simulink model "bscfsm"  (R2016a)
settings: Solver=FixedStepAuto  StartTime=0.0  StopTime=10  RelTol=1e-3
model workspace (MAT data in the model file):
  F = [0; 0; 0; 0; 0; 0; 0; 0; 0; 0; 0; 0; 0; 0; 0; 0; 0; 0; 0; 0; 0; 0; 0; 0; 0; 0; 0; 0; 0; 0; 0; 0; 0; 0; 0; 0; 0; 0; 0; 0; 0; 0; 0; 0; 0; 0; 0; 0; 0; 0; 0]
  FR = [0; 0; 0; 0; 0; 0]
  Ft = 0
  InputSize = 6
  M = [0 0 0 1 1 0 3 5.8]
  N = 32
  T = table
  T.nrows = 1
  T.nvars = 8
  T.varnames = {'Var1', 'Var2', 'Var3', 'Var4', 'Var5', 'Var6', 'Var7', 'Var8'}
  T.data = {0, 0, 0, 1, 1, 0, 3, 5.8}
  TimeSteps = 51
  X = [0 1 0 1 1 0 1 0 0.988521387031 1 1 0.0114786129688 ... (1224 elements, 6x204)]
  apfail = [0; 1; 0; 0.995818544823; 0; 0; 1; 0.00917624141749; 0.992109239838; 0; 0; 0.0226449188505; 0; 1; 1; 0; 0; 0.969073769871; 0; 0; 1; 0; 1; 1; 0.964844416339; 0; 1; 0; 0; 0; 1; 0; 0.982847610626; 1; 1; 1; 1; 1; 0; 1; 0; 1; 1; 0; 0.958770144702; 1; 1; 0; 1; 1; 0]
  cs : Simulink.ConfigSet (value not decoded)
  curPath = ''
  d = 52
  good = [0; 1; 1; 1; 1; 1; 1; 1; 1; 1; 1; 1; 1; 1; 1; 1; 1; 1; 1; 1; 1; 1; 1; 1; 1; 1; 1; 1; 1; 1; 1; 1; 1; 1; 1; 1; 1; 1; 1; 1; 1; 1; 1; 1; 1; 1; 1; 1; 1; 1; 1]
  hws : Simulink.ModelWorkspace (value not decoded)
  i = 14
  j = 51
  limits = [1; 0; 0; 0; 0; 0; 0; 1; 0; 1; 0.00163106788269; 1; 1; 1; 1; 0; 1; 0; 0; 1; 1; 0.0696477276458; 1; 1; 1; 0; 1; 0; 1; 1; 1; 0; 0.98345473187; 1; 0; 1; 1; 0.00166422824427; 0; 0; 1; 1; 0; 1; 0; 0; 0; 1; 0; 1; 1]
  list(1).name = 'F'
  list(1).size = [51 1]
  list(1).bytes = 408
  list(1).class = 'double'
  list(1).global = 0
  list(1).sparse = 0
  list(1).complex = 0
  list(1).nesting.function = 'simfsm'
  list(1).nesting.level = 1
  list(1).persistent = 0
  list(2).name = 'FR'
  list(2).size = [6 1]
  list(2).bytes = 48
  list(2).class = 'double'
  list(2).global = 0
  list(2).sparse = 0
  list(2).complex = 0
  list(2).nesting.function = 'simfsm'
  list(2).nesting.level = 1
  list(2).persistent = 0
  list(3).name = 'Ft'
  list(3).size = [1 1]
  list(3).bytes = 8
  list(3).class = 'double'
  list(3).global = 0
  list(3).sparse = 0
  list(3).complex = 0
  list(3).nesting.function = 'simfsm'
  list(3).nesting.level = 1
  list(3).persistent = 0
  list(4).name = 'InputSize'
  list(4).size = [1 1]
  list(4).bytes = 8
  list(4).class = 'double'
  list(4).global = 0
  list(4).sparse = 0
  list(4).complex = 0
  list(4).nesting.function = 'simfsm'
  list(4).nesting.level = 1
  list(4).persistent = 0
  list(5).name = 'N'
  list(5).size = [1 1]
  list(5).bytes = 8
  list(5).class = 'double'
  list(5).global = 0
  list(5).sparse = 0
  list(5).complex = 0
  list(5).nesting.function = 'simfsm'
  list(5).nesting.level = 1
  list(5).persistent = 0
  list(6).name = 'TimeSteps'
  list(6).size = [1 1]
  list(6).bytes = 8
  list(6).class = 'double'
  list(6).global = 0
  list(6).sparse = 0
  list(6).complex = 0
  list(6).nesting.function = 'simfsm'
  list(6).nesting.level = 1
  list(6).persistent = 0
  list(7).name = 'X'
  list(7).size = [6 204]
  list(7).bytes = 9792
  list(7).class = 'double'
  list(7).global = 0
  list(7).sparse = 0
  list(7).complex = 0
  list(7).nesting.function = 'simfsm'
  list(7).nesting.level = 1
  list(7).persistent = 0
  list(8).name = 'apfail'
  list(8).size = [51 1]
  list(8).bytes = 408
  list(8).class = 'double'
  list(8).global = 0
  list(8).sparse = 0
  list(8).complex = 0
  list(8).nesting.function = 'simfsm'
  list(8).nesting.level = 1
  list(8).persistent = 0
  list(9).name = 'cs'
  list(9).size = [1 1]
  list(9).bytes = 0
  list(9).class = 'Simulink.ConfigSet'
  list(9).global = 0
  list(9).sparse = 0
  list(9).complex = 0
  list(9).nesting.function = 'simfsm'
  list(9).nesting.level = 1
  list(9).persistent = 0
  list(10).name = 'curPath'
  list(10).size = [0 0]
  list(10).bytes = 0
  list(10).class = 'char'
  list(10).global = 0
  list(10).sparse = 0
  list(10).complex = 0
  list(10).nesting.function = 'simfsm'
  list(10).nesting.level = 1
  list(10).persistent = 0
  list(11).name = 'd'
  list(11).size = [1 1]
  list(11).bytes = 8
  list(11).class = 'double'
  list(11).global = 0
  list(11).sparse = 0
  list(11).complex = 0
  list(11).nesting.function = 'simfsm'
  list(11).nesting.level = 1
  list(11).persistent = 0
  list(12).name = 'good'
  list(12).size = [51 1]
  list(12).bytes = 51
  list(12).class = 'logical'
  list(12).global = 0
  list(12).sparse = 0
  list(12).complex = 0
  list(12).nesting.function = 'simfsm'
  list(12).nesting.level = 1
  list(12).persistent = 0
  list(13).name = 'hws'
  list(13).size = [1 1]
  list(13).bytes = 0
  list(13).class = 'Simulink.ModelWorkspace'
  list(13).global = 0
  list(13).sparse = 0
  list(13).complex = 0
  list(13).nesting.function = 'simfsm'
  list(13).nesting.level = 1
  list(13).persistent = 0
  list(14).name = 'i'
  list(14).size = [1 1]
  list(14).bytes = 8
  list(14).class = 'double'
  list(14).global = 0
  list(14).sparse = 0
  list(14).complex = 0
  list(14).nesting.function = 'simfsm'
  list(14).nesting.level = 1
  list(14).persistent = 0
  list(15).name = 'j'
  list(15).size = [1 1]
  list(15).bytes = 8
  list(15).class = 'double'
  list(15).global = 0
  list(15).sparse = 0
  list(15).complex = 0
  list(15).nesting.function = 'simfsm'
  list(15).nesting.level = 1
  list(15).persistent = 0
  list(16).name = 'limits'
  list(16).size = [51 1]
  list(16).bytes = 408
  list(16).class = 'double'
  list(16).global = 0
  list(16).sparse = 0
  list(16).complex = 0
  list(16).nesting.function = 'simfsm'
  list(16).nesting.level = 1
  list(16).persistent = 0
  list(17).name = 'list'
  list(17).size = [32 1]
  list(17).bytes = 46434
  list(17).class = 'struct'
  list(17).global = 0
  list(17).sparse = 0
  list(17).complex = 0
  list(17).nesting.function = 'simfsm'
  list(17).nesting.level = 1
  list(17).persistent = 0
  list(18).name = 'mode'
  list(18).size = [51 1]
  list(18).bytes = 51
  list(18).class = 'logical'
  list(18).global = 0
  list(18).sparse = 0
  list(18).complex = 0
  list(18).nesting.function = 'simfsm'
  list(18).nesting.level = 1
  list(18).persistent = 0
  list(19).name = 'model_cs'
  list(19).size = [1 1]
  list(19).bytes = 0
  list(19).class = 'Simulink.ConfigSet'
  list(19).global = 0
  list(19).sparse = 0
  list(19).complex = 0
  list(19).nesting.function = 'simfsm'
  list(19).nesting.level = 1
  list(19).persistent = 0
  list(20).name = 'modelpath'
  list(20).size = [0 0]
  list(20).bytes = 0
  list(20).class = 'char'
  list(20).global = 0
  list(20).sparse = 0
  list(20).complex = 0
  list(20).nesting.function = 'simfsm'
  list(20).nesting.level = 1
  list(20).persistent = 0
  list(21).name = 'n'
  list(21).size = [1 1]
  list(21).bytes = 8
  list(21).class = 'double'
  list(21).global = 0
  list(21).sparse = 0
  list(21).complex = 0
  list(21).nesting.function = 'simfsm'
  list(21).nesting.level = 1
  list(21).persistent = 0
  list(22).name = 'nbrInputs'
  list(22).size = [1 1]
  list(22).bytes = 8
  list(22).class = 'double'
  list(22).global = 0
  list(22).sparse = 0
  list(22).complex = 0
  list(22).nesting.function = 'simfsm'
  list(22).nesting.level = 1
  list(22).persistent = 0
  list(23).name = 'pullup'
  list(23).size = [51 1]
  list(23).bytes = 51
  list(23).class = 'logical'
  list(23).global = 0
  list(23).sparse = 0
  list(23).complex = 0
  list(23).nesting.function = 'simfsm'
  list(23).nesting.level = 1
  list(23).persistent = 0
  list(24).name = 'request'
  list(24).size = [51 1]
  list(24).bytes = 51
  list(24).class = 'logical'
  list(24).global = 0
  list(24).sparse = 0
  list(24).complex = 0
  list(24).nesting.function = 'simfsm'
  list(24).nesting.level = 1
  list(24).persistent = 0
  list(25).name = 'senstate'
  list(25).size = [51 1]
  list(25).bytes = 408
  list(25).class = 'double'
  list(25).global = 0
  list(25).sparse = 0
  list(25).complex = 0
  list(25).nesting.function = 'simfsm'
  list(25).nesting.level = 1
  list(25).persistent = 0
  list(26).name = 'simOut'
  list(26).size = [1 1]
  list(26).bytes = 34272
  list(26).class = 'Simulink.SimulationOutput'
  list(26).global = 0
  list(26).sparse = 0
  list(26).complex = 0
  list(26).nesting.function = 'simfsm'
  list(26).nesting.level = 1
  list(26).persistent = 0
  list(27).name = 'standby'
  list(27).size = [51 1]
  list(27).bytes = 408
  list(27).class = 'double'
  list(27).global = 0
  list(27).sparse = 0
  list(27).complex = 0
  list(27).nesting.function = 'simfsm'
  list(27).nesting.level = 1
  list(27).persistent = 0
  list(28).name = 'state'
  list(28).size = [51 1]
  list(28).bytes = 408
  list(28).class = 'double'
  list(28).global = 0
  list(28).sparse = 0
  list(28).complex = 0
  list(28).nesting.function = 'simfsm'
  list(28).nesting.level = 1
  list(28).persistent = 0
  list(29).name = 'supported'
  list(29).size = [51 1]
  list(29).bytes = 408
  list(29).class = 'double'
  list(29).global = 0
  list(29).sparse = 0
  list(29).complex = 0
  list(29).nesting.function = 'simfsm'
  list(29).nesting.level = 1
  list(29).persistent = 0
  list(30).name = 't'
  list(30).size = [51 1]
  list(30).bytes = 408
  list(30).class = 'double'
  list(30).global = 0
  list(30).sparse = 0
  list(30).complex = 0
  list(30).nesting.function = 'simfsm'
  list(30).nesting.level = 1
  list(30).persistent = 0
  list(31).name = 'var'
  list(31).size = [1 1]
  list(31).bytes = 3448
  list(31).class = 'struct'
  list(31).global = 0
  list(31).sparse = 0
  list(31).complex = 0
  list(31).nesting.function = 'simfsm'
  list(31).nesting.level = 1
  list(31).persistent = 0
  list(32).name = 'varout'
  list(32).size = [1 1]
  list(32).bytes = 4924
  list(32).class = 'struct'
  list(32).global = 0
  list(32).sparse = 0
  list(32).complex = 0
  list(32).nesting.function = 'simfsm'
  list(32).nesting.level = 1
  list(32).persistent = 0
  mode = [1; 1; 0; 1; 0; 1; 1; 0; 0; 1; 1; 1; 1; 1; 1; 1; 1; 1; 1; 0; 1; 1; 1; 1; 1; 1; 1; 1; 1; 1; 1; 1; 1; 1; 1; 1; 1; 1; 1; 1; 1; 1; 1; 0; 1; 1; 1; 1; 1; 1; 1]
  model_cs : Simulink.ConfigSet (value not decoded)
  modelpath = ''
  n = 6
  nbrInputs = 4
  nbrelements = 204
  pullup = [0; 1; 0; 0; 0; 0; 1; 0; 0; 0; 0; 1; 0; 1; 0; 0; 0; 1; 0; 0; 0; 0; 1; 0; 1; 1; 0; 0; 0; 1; 0; 1; 0; 1; 0; 1; 0; 1; 0; 1; 1; 0; 1; 0; 0; 1; 1; 1; 0; 1; 0]
  request = [0; 0; 1; 0; 1; 0; 0; 1; 1; 0; 0; 0; 0; 0; 0; 0; 0; 0; 0; 1; 0; 0; 0; 0; 0; 0; 0; 0; 0; 0; 0; 0; 0; 0; 0; 0; 0; 0; 0; 0; 0; 0; 0; 1; 0; 0; 0; 0; 0; 0; 0]
  senstate = [2; 1; 1; 1; 1; 1; 1; 1; 1; 1; 1; 1; 1; 1; 1; 1; 1; 1; 1; 1; 1; 1; 1; 1; 1; 1; 1; 1; 1; 1; 1; 1; 1; 1; 1; 1; 1; 1; 1; 1; 1; 1; 1; 1; 1; 1; 1; 1; 1; 1; 1]
  simOut = Simulink.SimulationOutput
  simOut.Data.tout = [0; 0.2; 0.4; 0.6; 0.8; 1; 1.2; 1.4; 1.6; 1.8; 2; 2.2; 2.4; 2.6; 2.8; 3; 3.2; 3.4; 3.6; 3.8; 4; 4.2; 4.4; 4.6; 4.8; 5; 5.2; 5.4; 5.6; 5.8; 6; 6.2; 6.4; 6.6; 6.8; 7; 7.2; 7.4; 7.6; 7.8; 8; 8.2; 8.4; 8.6; 8.8; 9; 9.2; 9.4; 9.6; 9.8; 10]
  simOut.Data.varout.time = [0; 0.2; 0.4; 0.6; 0.8; 1; 1.2; 1.4; 1.6; 1.8; 2; 2.2; 2.4; 2.6; 2.8; 3; 3.2; 3.4; 3.6; 3.8; 4; 4.2; 4.4; 4.6; 4.8; 5; 5.2; 5.4; 5.6; 5.8; 6; 6.2; 6.4; 6.6; 6.8; 7; 7.2; 7.4; 7.6; 7.8; 8; 8.2; 8.4; 8.6; 8.8; 9; 9.2; 9.4; 9.6; 9.8; 10]
  simOut.Data.varout.signals(1).values = [0; 1; 0; 0; 0; 0; 1; 0; 0; 0; 0; 1; 0; 1; 0; 0; 0; 1; 0; 0; 0; 0; 1; 0; 1; 1; 0; 0; 0; 1; 0; 1; 0; 1; 0; 1; 0; 1; 0; 1; 1; 0; 1; 0; 0; 1; 1; 1; 0; 1; 0]
  simOut.Data.varout.signals(1).dimensions = 1
  simOut.Data.varout.signals(1).label = ''
  simOut.Data.varout.signals(1).blockName = 'bscfsm/pullup'
  simOut.Data.varout.signals(2).values = [3; 2; 0; 3; 0; 3; 2; 0; 0; 3; 3; 2; 3; 2; 3; 3; 3; 2; 3; 0; 3; 3; 2; 3; 2; 2; 3; 3; 3; 2; 3; 2; 3; 2; 3; 2; 3; 2; 3; 2; 2; 3; 2; 0; 3; 2; 2; 2; 3; 2; 3]
  simOut.Data.varout.signals(2).dimensions = 1
  simOut.Data.varout.signals(2).label = ''
  simOut.Data.varout.signals(2).blockName = 'bscfsm/state'
  simOut.Data.varout.signals(3).values = [0; 1; 1; 1; 1; 1; 1; 1; 1; 1; 1; 1; 1; 1; 1; 1; 1; 1; 1; 1; 1; 1; 1; 1; 1; 1; 1; 1; 1; 1; 1; 1; 1; 1; 1; 1; 1; 1; 1; 1; 1; 1; 1; 1; 1; 1; 1; 1; 1; 1; 1]
  simOut.Data.varout.signals(3).dimensions = 1
  simOut.Data.varout.signals(3).label = ''
  simOut.Data.varout.signals(3).blockName = 'bscfsm/good'
  simOut.Data.varout.signals(4).values = [2; 1; 1; 1; 1; 1; 1; 1; 1; 1; 1; 1; 1; 1; 1; 1; 1; 1; 1; 1; 1; 1; 1; 1; 1; 1; 1; 1; 1; 1; 1; 1; 1; 1; 1; 1; 1; 1; 1; 1; 1; 1; 1; 1; 1; 1; 1; 1; 1; 1; 1]
  simOut.Data.varout.signals(4).dimensions = 1
  simOut.Data.varout.signals(4).label = ''
  simOut.Data.varout.signals(4).blockName = 'bscfsm/SENSTATE'
  simOut.Data.varout.signals(5).values = [1; 1; 0; 1; 0; 1; 1; 0; 0; 1; 1; 1; 1; 1; 1; 1; 1; 1; 1; 0; 1; 1; 1; 1; 1; 1; 1; 1; 1; 1; 1; 1; 1; 1; 1; 1; 1; 1; 1; 1; 1; 1; 1; 0; 1; 1; 1; 1; 1; 1; 1]
  simOut.Data.varout.signals(5).dimensions = 1
  simOut.Data.varout.signals(5).label = ''
  simOut.Data.varout.signals(5).blockName = 'bscfsm/MODE'
  simOut.Data.varout.signals(6).values = [0; 0; 1; 0; 1; 0; 0; 1; 1; 0; 0; 0; 0; 0; 0; 0; 0; 0; 0; 1; 0; 0; 0; 0; 0; 0; 0; 0; 0; 0; 0; 0; 0; 0; 0; 0; 0; 0; 0; 0; 0; 0; 0; 1; 0; 0; 0; 0; 0; 0; 0]
  simOut.Data.varout.signals(6).dimensions = 1
  simOut.Data.varout.signals(6).label = ''
  simOut.Data.varout.signals(6).blockName = 'bscfsm/REQUEST'
  simOut.Metadata = Simulink.SimulationMetadata
  simOut.Metadata.ModelInfo.ModelName = 'bscfsm'
  simOut.Metadata.ModelInfo.ModelVersion = '1.101'
  simOut.Metadata.ModelInfo.ModelFilePath = '/Users/ceren.gebizli/Desktop/Shiva/QRA-Search/QRA-Search/SimulinkModels/1_fsm/bscfsm.slx'
  simOut.Metadata.ModelInfo.UserID = 'ceren.gebizli'
  simOut.Metadata.ModelInfo.MachineName = ''
  simOut.Metadata.ModelInfo.Platform = 'MACI64'
  simOut.Metadata.ModelInfo.ModelStructuralChecksum = [2182324134; 966261521; 1592501320; 2819510478]
  simOut.Metadata.ModelInfo.SimulationMode = 'normal'
  simOut.Metadata.ModelInfo.StartTime = 0
  simOut.Metadata.ModelInfo.StopTime = 10
  simOut.Metadata.ModelInfo.SolverInfo.Type = 'Fixed-Step'
  simOut.Metadata.ModelInfo.SolverInfo.Solver = 'FixedStepDiscrete'
  simOut.Metadata.ModelInfo.SolverInfo.FixedStepSize = 0.2
  simOut.Metadata.ModelInfo.SimulinkVersion.Name = 'Simulink'
  simOut.Metadata.ModelInfo.SimulinkVersion.Version = '8.7'
  simOut.Metadata.ModelInfo.SimulinkVersion.Release = '(R2016a)'
  simOut.Metadata.ModelInfo.SimulinkVersion.Date = '10-Feb-2016'
  simOut.Metadata.TimingInfo.WallClockTimestampStart = '2018-04-07 19:41:48.010033'
  simOut.Metadata.TimingInfo.WallClockTimestampStop = '2018-04-07 19:41:48.615294'
  simOut.Metadata.TimingInfo.InitializationElapsedWallTime = 0.5552
  simOut.Metadata.TimingInfo.ExecutionElapsedWallTime = 0.000757
  simOut.Metadata.TimingInfo.TerminationElapsedWallTime = 0.049317
  simOut.Metadata.TimingInfo.TotalElapsedWallTime = 0.605274
  simOut.Metadata.ExecutionInfo.StopEvent = 'ReachedStopTime'
  simOut.Metadata.ExecutionInfo.StopEventSource = []
  simOut.Metadata.ExecutionInfo.StopEventDescription = 'Reached stop time of 10'
  simOut.Metadata.ExecutionInfo.ErrorDiagnostic = []
  simOut.Metadata.ExecutionInfo.WarningDiagnostics(1).Diagnostic = MSLDiagnostic
  simOut.Metadata.ExecutionInfo.WarningDiagnostics(1).Diagnostic.identifier = 'Simulink:blocks:MatchingFromNotFound'
  simOut.Metadata.ExecutionInfo.WarningDiagnostics(1).Diagnostic.message = 'Matching "From" for "Goto" ''<a href="matlab:open_and_hilite_hyperlink (''bscfsm/FiniteStateMachine/Manager/Actions/Maneuver/Goto1'',''error'')">bscfsm/FiniteStateMachine/Manager/Actions/Maneuver/Goto1</a>'' not found'
  simOut.Metadata.ExecutionInfo.WarningDiagnostics(1).Diagnostic.paths = {'bscfsm/FiniteStateMachine/Manager/Actions/Maneuver/Goto1'}
  simOut.Metadata.ExecutionInfo.WarningDiagnostics(1).Diagnostic.arguments = {'bscfsm/FiniteStateMachine/Manager/Actions/Maneuver/Goto1'}
  simOut.Metadata.ExecutionInfo.WarningDiagnostics(1).SimulationPhase = 'Initialization'
  simOut.Metadata.ExecutionInfo.WarningDiagnostics(1).SimulationTime = []
  simOut.Metadata.ExecutionInfo.WarningDiagnostics(2).Diagnostic = MSLDiagnostic
  simOut.Metadata.ExecutionInfo.WarningDiagnostics(2).Diagnostic.identifier = 'Simulink:blocks:BlockWithFewExplicitICsFeedingEmptyOutportConsistentOutportInit'
  simOut.Metadata.ExecutionInfo.WarningDiagnostics(2).Diagnostic.message = 'The initial output of Outport ''<a href="matlab:open_and_hilite_hyperlink (''bscfsm/FiniteStateMachine/Manager/Output/Maneuver/Output'',''error'')">bscfsm/FiniteStateMachine/Manager/Output/Maneuver/Output</a>'' is set to [] which might cause unexpected initialization. If you want output port 1 of Subsystem ''<a href="matlab:open_and_hilite_hyperlink (''bscfsm/FiniteStateMachine/Manager/Output/Maneuver'',''error'')">bscfsm/FiniteStateMachine/Manager/Output/Maneuver</a>'' to have the same initial value as the Outport sources, ''bscfsm/FiniteStateMachine/Manager/Output/Maneuver/Constant9'', ''bscfsm/FiniteStateMachine/Manager/Output/Maneuver/Constant11'', ''bscfsm/FiniteStateMachine/Manager/Output/Maneuver/Constant10'', please explicitly set this initial output value on ''<a href="matlab:open_and_hilite_hyperlink (''bscfsm/FiniteStateMachine/Manager/Output/Maneuver/Output'',''error'')">bscfsm/FiniteStateMachine/Manager/Output/Maneuver/Output</a>''. To turn off this warning message, deselect <a href="matlab:load_system(''bscfsm/FiniteStateMachine/Manager/Output/Maneuver/Output'');configset.highlightParameter(''bscfsm/FiniteStateMachine/Manager/Output/Maneuver/Output'',''CheckSSInitialOutputMsg'');">Check undefined subsystem initial output</a>.'
  simOut.Metadata.ExecutionInfo.WarningDiagnostics(2).Diagnostic.paths = {'bscfsm/FiniteStateMachine/Manager/Output/Maneuver/Output', 'bscfsm/FiniteStateMachine/Manager/Output/Maneuver', 'bscfsm/FiniteStateMachine/Manager/Output/Maneuver/Output'}
  simOut.Metadata.ExecutionInfo.WarningDiagnostics(2).Diagnostic.arguments = {'bscfsm/FiniteStateMachine/Manager/Output/Maneuver/Output', 1, 'bscfsm/FiniteStateMachine/Manager/Output/Maneuver', '''bscfsm/FiniteStateMachine/Manager/Output/Maneuver/Constant9'', ''bscfsm/FiniteStateMachine/Manager/Output/Maneuver/Constant11'', ''bscfsm/FiniteStateMachine/Manager/Output/Maneuver/Constant10''', 'bscfsm/FiniteStateMachine/Manager/Output/Maneuver/Output'}
  simOut.Metadata.ExecutionInfo.WarningDiagnostics(2).SimulationPhase = 'Initialization'
  simOut.Metadata.ExecutionInfo.WarningDiagnostics(2).SimulationTime = []
  simOut.Metadata.ExecutionInfo.WarningDiagnostics(3).Diagnostic = MSLDiagnostic
  simOut.Metadata.ExecutionInfo.WarningDiagnostics(3).Diagnostic.identifier = 'Simulink:blocks:BlockWithFewExplicitICsFeedingEmptyOutportConsistentOutportInit'
  simOut.Metadata.ExecutionInfo.WarningDiagnostics(3).Diagnostic.message = 'The initial output of Outport ''<a href="matlab:open_and_hilite_hyperlink (''bscfsm/FiniteStateMachine/Manager/Output/Nominal/Output'',''error'')">bscfsm/FiniteStateMachine/Manager/Output/Nominal/Output</a>'' is set to [] which might cause unexpected initialization. If you want output port 1 of Subsystem ''<a href="matlab:open_and_hilite_hyperlink (''bscfsm/FiniteStateMachine/Manager/Output/Nominal'',''error'')">bscfsm/FiniteStateMachine/Manager/Output/Nominal</a>'' to have the same initial value as the Outport sources, ''bscfsm/FiniteStateMachine/Manager/Output/Nominal/Constant4'', ''bscfsm/FiniteStateMachine/Manager/Output/Nominal/Constant5'', ''bscfsm/FiniteStateMachine/Manager/Output/Nominal/Constant3'', please explicitly set this initial output value on ''<a href="matlab:open_and_hilite_hyperlink (''bscfsm/FiniteStateMachine/Manager/Output/Nominal/Output'',''error'')">bscfsm/FiniteStateMachine/Manager/Output/Nominal/Output</a>''. To turn off this warning message, deselect <a href="matlab:load_system(''bscfsm/FiniteStateMachine/Manager/Output/Nominal/Output'');configset.highlightParameter(''bscfsm/FiniteStateMachine/Manager/Output/Nominal/Output'',''CheckSSInitialOutputMsg'');">Check undefined subsystem initial output</a>.'
  simOut.Metadata.ExecutionInfo.WarningDiagnostics(3).Diagnostic.paths = {'bscfsm/FiniteStateMachine/Manager/Output/Nominal/Output', 'bscfsm/FiniteStateMachine/Manager/Output/Nominal', 'bscfsm/FiniteStateMachine/Manager/Output/Nominal/Output'}
  simOut.Metadata.ExecutionInfo.WarningDiagnostics(3).Diagnostic.arguments = {'bscfsm/FiniteStateMachine/Manager/Output/Nominal/Output', 1, 'bscfsm/FiniteStateMachine/Manager/Output/Nominal', '''bscfsm/FiniteStateMachine/Manager/Output/Nominal/Constant4'', ''bscfsm/FiniteStateMachine/Manager/Output/Nominal/Constant5'', ''bscfsm/FiniteStateMachine/Manager/Output/Nominal/Constant3''', 'bscfsm/FiniteStateMachine/Manager/Output/Nominal/Output'}
  simOut.Metadata.ExecutionInfo.WarningDiagnostics(3).SimulationPhase = 'Initialization'
  simOut.Metadata.ExecutionInfo.WarningDiagnostics(3).SimulationTime = []
  simOut.Metadata.ExecutionInfo.WarningDiagnostics(4).Diagnostic = MSLDiagnostic
  simOut.Metadata.ExecutionInfo.WarningDiagnostics(4).Diagnostic.identifier = 'Simulink:blocks:BlockWithFewExplicitICsFeedingEmptyOutportConsistentOutportInit'
  simOut.Metadata.ExecutionInfo.WarningDiagnostics(4).Diagnostic.message = 'The initial output of Outport ''<a href="matlab:open_and_hilite_hyperlink (''bscfsm/FiniteStateMachine/Manager/Output/Standby/Output'',''error'')">bscfsm/FiniteStateMachine/Manager/Output/Standby/Output</a>'' is set to [] which might cause unexpected initialization. If you want output port 1 of Subsystem ''<a href="matlab:open_and_hilite_hyperlink (''bscfsm/FiniteStateMachine/Manager/Output/Standby'',''error'')">bscfsm/FiniteStateMachine/Manager/Output/Standby</a>'' to have the same initial value as the Outport sources, ''bscfsm/FiniteStateMachine/Manager/Output/Standby/Constant9'', ''bscfsm/FiniteStateMachine/Manager/Output/Standby/Constant11'', ''bscfsm/FiniteStateMachine/Manager/Output/Standby/Constant1'', please explicitly set this initial output value on ''<a href="matlab:open_and_hilite_hyperlink (''bscfsm/FiniteStateMachine/Manager/Output/Standby/Output'',''error'')">bscfsm/FiniteStateMachine/Manager/Output/Standby/Output</a>''. To turn off this warning message, deselect <a href="matlab:load_system(''bscfsm/FiniteStateMachine/Manager/Output/Standby/Output'');configset.highlightParameter(''bscfsm/FiniteStateMachine/Manager/Output/Standby/Output'',''CheckSSInitialOutputMsg'');">Check undefined subsystem initial output</a>.'
  simOut.Metadata.ExecutionInfo.WarningDiagnostics(4).Diagnostic.paths = {'bscfsm/FiniteStateMachine/Manager/Output/Standby/Output', 'bscfsm/FiniteStateMachine/Manager/Output/Standby', 'bscfsm/FiniteStateMachine/Manager/Output/Standby/Output'}
  simOut.Metadata.ExecutionInfo.WarningDiagnostics(4).Diagnostic.arguments = {'bscfsm/FiniteStateMachine/Manager/Output/Standby/Output', 1, 'bscfsm/FiniteStateMachine/Manager/Output/Standby', '''bscfsm/FiniteStateMachine/Manager/Output/Standby/Constant9'', ''bscfsm/FiniteStateMachine/Manager/Output/Standby/Constant11'', ''bscfsm/FiniteStateMachine/Manager/Output/Standby/Constant1''', 'bscfsm/FiniteStateMachine/Manager/Output/Standby/Output'}
  simOut.Metadata.ExecutionInfo.WarningDiagnostics(4).SimulationPhase = 'Initialization'
  simOut.Metadata.ExecutionInfo.WarningDiagnostics(4).SimulationTime = []
  simOut.Metadata.ExecutionInfo.WarningDiagnostics(5).Diagnostic = MSLDiagnostic
  simOut.Metadata.ExecutionInfo.WarningDiagnostics(5).Diagnostic.identifier = 'Simulink:blocks:BlockWithFewExplicitICsFeedingEmptyOutportConsistentOutportInit'
  simOut.Metadata.ExecutionInfo.WarningDiagnostics(5).Diagnostic.message = 'The initial output of Outport ''<a href="matlab:open_and_hilite_hyperlink (''bscfsm/FiniteStateMachine/Manager/Output/Transition/Output'',''error'')">bscfsm/FiniteStateMachine/Manager/Output/Transition/Output</a>'' is set to [] which might cause unexpected initialization. If you want output port 1 of Subsystem ''<a href="matlab:open_and_hilite_hyperlink (''bscfsm/FiniteStateMachine/Manager/Output/Transition'',''error'')">bscfsm/FiniteStateMachine/Manager/Output/Transition</a>'' to have the same initial value as the Outport sources, ''bscfsm/FiniteStateMachine/Manager/Output/Transition/Constant18'', ''bscfsm/FiniteStateMachine/Manager/Output/Transition/Constant17'', ''bscfsm/FiniteStateMachine/Manager/Output/Transition/Constant16'', please explicitly set this initial output value on ''<a href="matlab:open_and_hilite_hyperlink (''bscfsm/FiniteStateMachine/Manager/Output/Transition/Output'',''error'')">bscfsm/FiniteStateMachine/Manager/Output/Transition/Output</a>''. To turn off this warning message, deselect <a href="matlab:load_system(''bscfsm/FiniteStateMachine/Manager/Output/Transition/Output'');configset.highlightParameter(''bscfsm/FiniteStateMachine/Manager/Output/Transition/Output'',''CheckSSInitialOutputMsg'');">Check undefined subsystem initial output</a>.'
  simOut.Metadata.ExecutionInfo.WarningDiagnostics(5).Diagnostic.paths = {'bscfsm/FiniteStateMachine/Manager/Output/Transition/Output', 'bscfsm/FiniteStateMachine/Manager/Output/Transition', 'bscfsm/FiniteStateMachine/Manager/Output/Transition/Output'}
  simOut.Metadata.ExecutionInfo.WarningDiagnostics(5).Diagnostic.arguments = {'bscfsm/FiniteStateMachine/Manager/Output/Transition/Output', 1, 'bscfsm/FiniteStateMachine/Manager/Output/Transition', '''bscfsm/FiniteStateMachine/Manager/Output/Transition/Constant18'', ''bscfsm/FiniteStateMachine/Manager/Output/Transition/Constant17'', ''bscfsm/FiniteStateMachine/Manager/Output/Transition/Constant16''', 'bscfsm/FiniteStateMachine/Manager/Output/Transition/Output'}
  simOut.Metadata.ExecutionInfo.WarningDiagnostics(5).SimulationPhase = 'Initialization'
  simOut.Metadata.ExecutionInfo.WarningDiagnostics(5).SimulationTime = []
  simOut.Metadata.ExecutionInfo.WarningDiagnostics(6).Diagnostic = MSLDiagnostic
  simOut.Metadata.ExecutionInfo.WarningDiagnostics(6).Diagnostic.identifier = 'Simulink:SampleTime:FixedStepSizeHeuristicWarn'
  simOut.Metadata.ExecutionInfo.WarningDiagnostics(6).Diagnostic.message = 'Unable to determine a fixed step size based on the sample times in the model ''<a href="matlab:open_system (''bscfsm'')">bscfsm</a>'', because the model does not have any discrete sample times.  Picking a fixed step size of (0.2) based on simulation start and stop times.  You can disable this diagnostic by explicitly specifying a fixed step size in the Solver pane of the Configuration Parameters dialog box, or setting the ''Automatic solver parameter selection'' diagnostic to ''none'' in the Solver group on the Diagnostics pane of the Configuration Parameters dialog box.'
  simOut.Metadata.ExecutionInfo.WarningDiagnostics(6).Diagnostic.paths = {'bscfsm'}
  simOut.Metadata.ExecutionInfo.WarningDiagnostics(6).Diagnostic.arguments = {'bscfsm', '0.2'}
  simOut.Metadata.ExecutionInfo.WarningDiagnostics(6).SimulationPhase = 'Initialization'
  simOut.Metadata.ExecutionInfo.WarningDiagnostics(6).SimulationTime = []
  simOut.Metadata.AppInfo = struct()
  standby = [1; 1; 0; 0.989636007632; 0; 1; 0; 0; 0; 1; 1; 1; 1; 1; 1; 1; 1; 1; 1; 0; 1; 1; 0; 0.0394523699092; 0; 0; 1; 0; 0.965449367452; 0; 1; 1; 1; 0.936858086742; 0; 1; 1; 1; 1; 1; 0; 0.991326615097; 1; 0; 0.00279093512947; 0; 0; 0; 1; 0; 1]
  state = [3; 2; 0; 3; 0; 3; 2; 0; 0; 3; 3; 2; 3; 2; 3; 3; 3; 2; 3; 0; 3; 3; 2; 3; 2; 2; 3; 3; 3; 2; 3; 2; 3; 2; 3; 2; 3; 2; 3; 2; 2; 3; 2; 0; 3; 2; 2; 2; 3; 2; 3]
  supported = [0.987301836266; 1; 1; 0; 0.99444787553; 0; 0; 1; 0; 1; 1; 0; 0; 0.947955706868; 0.0127120599082; 0; 0.998670951305; 0; 0; 0; 0; 0.994963861004; 0.992716916569; 0; 1; 0; 0; 1; 1; 0; 0; 0; 1; 1; 1; 1; 1; 1; 1; 0; 0; 0; 0; 1; 0; 0.000620556033995; 0; 0; 1; 0; 0.969918687835]
  t = [0; 0.2; 0.4; 0.6; 0.8; 1; 1.2; 1.4; 1.6; 1.8; 2; 2.2; 2.4; 2.6; 2.8; 3; 3.2; 3.4; 3.6; 3.8; 4; 4.2; 4.4; 4.6; 4.8; 5; 5.2; 5.4; 5.6; 5.8; 6; 6.2; 6.4; 6.6; 6.8; 7; 7.2; 7.4; 7.6; 7.8; 8; 8.2; 8.4; 8.6; 8.8; 9; 9.2; 9.4; 9.6; 9.8; 10]
  var.time = [0 0.2 0.4 0.6 0.8 1 1.2 1.4 1.6 1.8 2 2.2 2.4 2.6 2.8 3 3.2 3.4 3.6 3.8 4 4.2 4.4 4.6 4.8 5 5.2 5.4 5.6 5.8 6 6.2 6.4 6.6 6.8 7 7.2 7.4 7.6 7.8 8 8.2 8.4 8.6 8.8 9 9.2 9.4 9.6 9.8 10]
  var.signals(1).values = [0; 0.0114786129688; 0; 0; 1; 1; 0; 0; 0.0410321784927; 0; 1; 1; 1; 0; 0; 0.998789229167; 0.990387240665; 0; 1; 0; 0; 1; 1; 0.00413955541821; 1; 1; 1; 0; 0; 0; 1; 1; 1; 0; 0; 0; 0; 1; 1; 0; 0.0172772443089; 0; 1; 0; 0; 1; 0; 0; 1; 1; 1]
  var.signals(1).dimensions = 1
  var.signals(2).values = [0; 0; 1; 1; 0; 1; 0; 1; 0; 0.986477065133; 1; 1; 0.994344328304; 0; 0; 0; 0; 0; 0; 0; 1; 0; 0; 0; 1; 1; 0; 1; 1; 1; 1; 0; 1; 1; 0; 1; 0; 1; 0; 0; 0; 0.967855142515; 1; 0; 0; 1; 0.0183628868839; 1; 1; 0; 0.0146452896222]
  var.signals(2).dimensions = 1
  var.signals(3).values = [1; 0; 0; 1; 1; 0; 0; 1; 0.0183702490806; 0; 0; 0; 1; 1; 1; 0.971162839334; 1; 0; 0.00188352841176; 1; 0; 1; 0; 1; 1; 0; 0.0295171611471; 0; 1; 1; 0.996206182332; 1; 0; 0; 0; 1; 0; 0; 0.980341786823; 1; 1; 0.93213779696; 1; 0; 1; 0; 0.992336790178; 1; 0; 1; 0]
  var.signals(3).dimensions = 1
  var.signals(4).values = [1; 1; 0; 0; 1; 1; 0; 0; 0; 0; 0; 1; 0; 1; 1; 0; 1; 0; 1; 1; 1; 1; 0; 0; 0; 0.996639893522; 0; 0.939532694751; 0; 0; 1; 1; 0; 1; 1; 0.838341649142; 0; 1; 0; 0.979204943341; 1; 1; 0; 0; 0; 0.00418789108046; 1; 0.0135071722538; 0.0267586516864; 0; 1]
  var.signals(4).dimensions = 1
  varout.time = [0; 0.2; 0.4; 0.6; 0.8; 1; 1.2; 1.4; 1.6; 1.8; 2; 2.2; 2.4; 2.6; 2.8; 3; 3.2; 3.4; 3.6; 3.8; 4; 4.2; 4.4; 4.6; 4.8; 5; 5.2; 5.4; 5.6; 5.8; 6; 6.2; 6.4; 6.6; 6.8; 7; 7.2; 7.4; 7.6; 7.8; 8; 8.2; 8.4; 8.6; 8.8; 9; 9.2; 9.4; 9.6; 9.8; 10]
  varout.signals(1).values = [0; 1; 0; 0; 0; 0; 1; 0; 0; 0; 0; 1; 0; 1; 0; 0; 0; 1; 0; 0; 0; 0; 1; 0; 1; 1; 0; 0; 0; 1; 0; 1; 0; 1; 0; 1; 0; 1; 0; 1; 1; 0; 1; 0; 0; 1; 1; 1; 0; 1; 0]
  varout.signals(1).dimensions = 1
  varout.signals(1).label = ''
  varout.signals(1).blockName = 'bscfsm/pullup'
  varout.signals(2).values = [3; 2; 0; 3; 0; 3; 2; 0; 0; 3; 3; 2; 3; 2; 3; 3; 3; 2; 3; 0; 3; 3; 2; 3; 2; 2; 3; 3; 3; 2; 3; 2; 3; 2; 3; 2; 3; 2; 3; 2; 2; 3; 2; 0; 3; 2; 2; 2; 3; 2; 3]
  varout.signals(2).dimensions = 1
  varout.signals(2).label = ''
  varout.signals(2).blockName = 'bscfsm/state'
  varout.signals(3).values = [0; 1; 1; 1; 1; 1; 1; 1; 1; 1; 1; 1; 1; 1; 1; 1; 1; 1; 1; 1; 1; 1; 1; 1; 1; 1; 1; 1; 1; 1; 1; 1; 1; 1; 1; 1; 1; 1; 1; 1; 1; 1; 1; 1; 1; 1; 1; 1; 1; 1; 1]
  varout.signals(3).dimensions = 1
  varout.signals(3).label = ''
  varout.signals(3).blockName = 'bscfsm/good'
  varout.signals(4).values = [2; 1; 1; 1; 1; 1; 1; 1; 1; 1; 1; 1; 1; 1; 1; 1; 1; 1; 1; 1; 1; 1; 1; 1; 1; 1; 1; 1; 1; 1; 1; 1; 1; 1; 1; 1; 1; 1; 1; 1; 1; 1; 1; 1; 1; 1; 1; 1; 1; 1; 1]
  varout.signals(4).dimensions = 1
  varout.signals(4).label = ''
  varout.signals(4).blockName = 'bscfsm/SENSTATE'
  varout.signals(5).values = [1; 1; 0; 1; 0; 1; 1; 0; 0; 1; 1; 1; 1; 1; 1; 1; 1; 1; 1; 0; 1; 1; 1; 1; 1; 1; 1; 1; 1; 1; 1; 1; 1; 1; 1; 1; 1; 1; 1; 1; 1; 1; 1; 0; 1; 1; 1; 1; 1; 1; 1]
  varout.signals(5).dimensions = 1
  varout.signals(5).label = ''
  varout.signals(5).blockName = 'bscfsm/MODE'
  varout.signals(6).values = [0; 0; 1; 0; 1; 0; 0; 1; 1; 0; 0; 0; 0; 0; 0; 0; 0; 0; 0; 1; 0; 0; 0; 0; 0; 0; 0; 0; 0; 0; 0; 0; 0; 0; 0; 0; 0; 0; 0; 0; 0; 0; 0; 1; 0; 0; 0; 0; 0; 0; 0]
  varout.signals(6).dimensions = 1
  varout.signals(6).label = ''
  varout.signals(6).blockName = 'bscfsm/REQUEST'
settings Model: Creator=elliocm  LastModifiedBy=ceren.gebizli
settings DataIOCC: ExternalInput=var  LimitDataPoints=on  LoadExternalInput=on  SaveFormat=StructureWithTime
settings OptimizationCC: ExpressionDepthLimit=2147483647
settings DebuggingCC: UnderspecifiedInitializationDetection=Classic  MergeDetectMultiDrivingBlocksExec=none  SolverPrmCheckMsg=warning  StateNameClashWarn=warning
settings HardwareCC: ProdBitPerPointer=32  ProdLargestAtomicFloat=None  ProdIntDivRoundTo=Undefined  ProdEndianess=Unspecified  ProdWordSize=32  ProdHWDeviceType=32-bit Generic
settings ModelReferenceCC: PropagateSignalLabelsOutOfModel=off
settings ConfigComp: CovModelRefEnable=Off

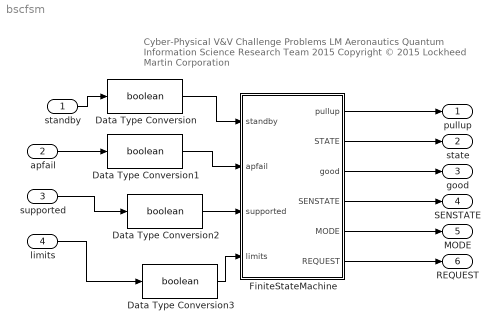
== system bscfsm ==
  note: Cyber-Physical V&V Challenge Problems
      | LM Aeronautics Quantum Information Science Research Team 2015
      | Copyright © 2015 Lockheed Martin Corporation
  standby : Inport  OutDataTypeStr=double
  apfail : Inport  Port=2  OutDataTypeStr=double
  supported : Inport  Port=3  OutDataTypeStr=double
  limits : Inport  Port=4  OutDataTypeStr=double
  Data Type Conversion{,1..3} (4 alike) : DataTypeConversion  OutDataTypeStr=boolean  RndMeth=Round
  FiniteStateMachine : Subsystem
  pullup : Outport
  state : Outport  Port=2
  good : Outport  Port=3
  SENSTATE : Outport  Port=4
  MODE : Outport  Port=5
  REQUEST : Outport  Port=6
  wires:
  FiniteStateMachine/1(pullup) -> pullup/1
  FiniteStateMachine/2(STATE) -> state/1
  FiniteStateMachine/3(good) -> good/1
  FiniteStateMachine/4(SENSTATE) -> SENSTATE/1
  FiniteStateMachine/5(MODE) -> MODE/1
  FiniteStateMachine/6(REQUEST) -> REQUEST/1
  standby/1 -> Data Type Conversion/1
  Data Type Conversion/1 -> FiniteStateMachine/1(standby)
  apfail/1 -> Data Type Conversion1/1
  Data Type Conversion1/1 -> FiniteStateMachine/2(apfail)
  Data Type Conversion2/1 -> FiniteStateMachine/3(supported)
  supported/1 -> Data Type Conversion2/1
  limits/1 -> Data Type Conversion3/1
  Data Type Conversion3/1 -> FiniteStateMachine/4(limits)

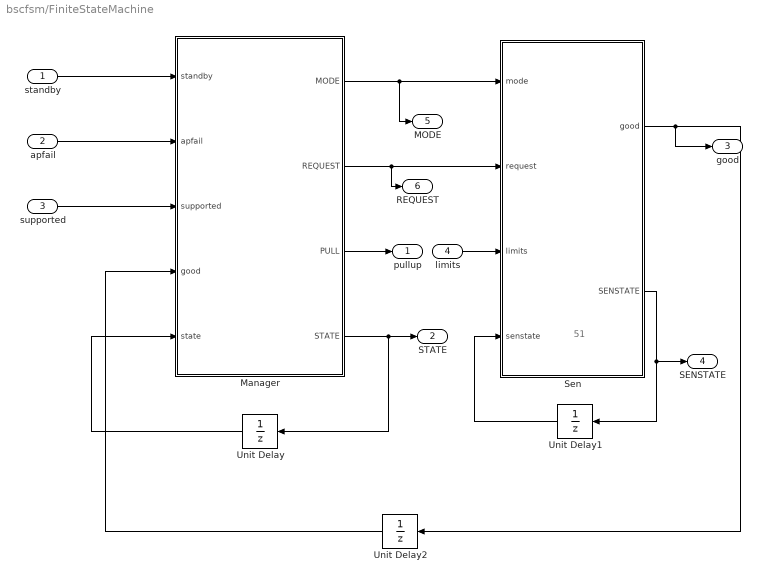
== system bscfsm/FiniteStateMachine ==
  note: 51
  standby : Inport
  apfail : Inport  Port=2
  supported : Inport  Port=3
  limits : Inport  Port=4
  Manager : Subsystem
  Sen : Subsystem
  Unit Delay : UnitDelay  SampleTime=-1
  Unit Delay1 : UnitDelay  SampleTime=-1
  Unit Delay2 : UnitDelay  InitialCondition=1  SampleTime=-1
  pullup : Outport
  STATE : Outport  Port=2
  good : Outport  Port=3
  SENSTATE : Outport  Port=4
  MODE : Outport  Port=5
  REQUEST : Outport  Port=6
  wires:
  Manager/1(MODE) -> MODE/1, Sen/1(mode)
  Manager/4(STATE) -> STATE/1, Unit Delay/1
  Manager/2(REQUEST) -> REQUEST/1, Sen/2(request)
  Unit Delay1/1 -> Sen/4(senstate)
  Unit Delay2/1 -> Manager/4(good)
  Sen/2(SENSTATE) -> SENSTATE/1, Unit Delay1/1
  Sen/1(good) -> good/1, Unit Delay2/1
  Manager/3(PULL) -> pullup/1
  standby/1 -> Manager/1(standby)
  apfail/1 -> Manager/2(apfail)
  supported/1 -> Manager/3(supported)
  limits/1 -> Sen/3(limits)
  Unit Delay/1 -> Manager/5(state)

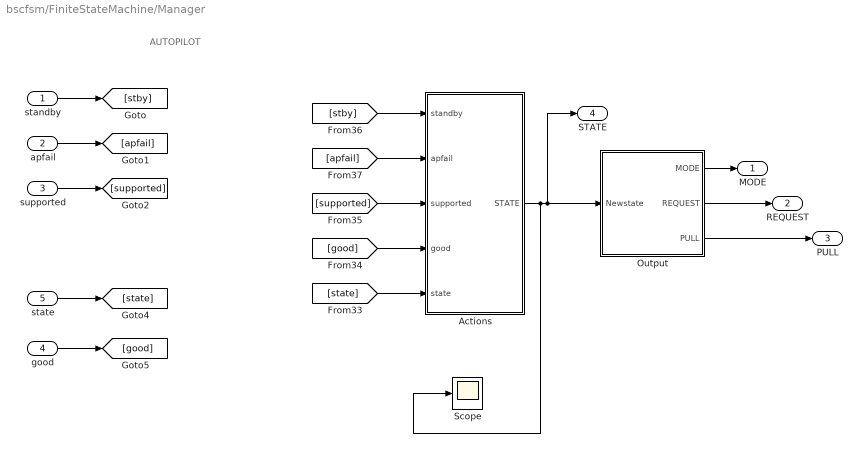
== system bscfsm/FiniteStateMachine/Manager ==
  note: AUTOPILOT
  standby : Inport
  apfail : Inport  Port=2
  supported : Inport  Port=3
  good : Inport  Port=4
  state : Inport  Port=5
  Actions : Subsystem
  Output : Subsystem
  Scope : Scope
  MODE : Outport
  REQUEST : Outport  Port=2
  PULL : Outport  Port=3
  STATE : Outport  Port=4
  wires:
  standby/1 -> [stby]
  supported/1 -> [supported]
  apfail/1 -> [apfail]
  state/1 -> [state]
  good/1 -> [good]
  Actions/1(STATE) -> Scope/1, Output/1(Newstate), STATE/1
  [apfail] -> Actions/2(apfail)
  [state] -> Actions/5(state)
  [supported] -> Actions/3(supported)
  [good] -> Actions/4(good)
  [stby] -> Actions/1(standby)
  Output/1(MODE) -> MODE/1
  Output/2(REQUEST) -> REQUEST/1
  Output/3(PULL) -> PULL/1

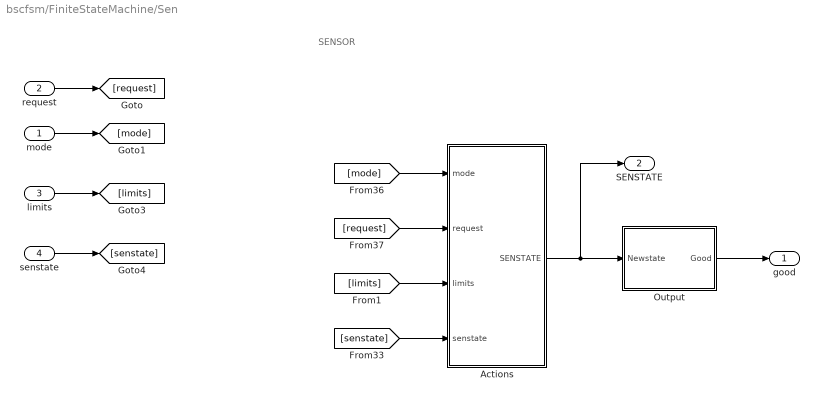
== system bscfsm/FiniteStateMachine/Sen ==
  note: SENSOR
  mode : Inport
  request : Inport  Port=2
  limits : Inport  Port=3
  senstate : Inport  Port=4
  Actions : Subsystem
  Output : Subsystem
  good : Outport
  SENSTATE : Outport  Port=2
  wires:
  request/1 -> [request]
  mode/1 -> [mode]
  limits/1 -> [limits]
  senstate/1 -> [senstate]
  Output/1(Good) -> good/1
  [request] -> Actions/2(request)
  [mode] -> Actions/1(mode)
  Actions/1(SENSTATE) -> Output/1(Newstate), SENSTATE/1
  [senstate] -> Actions/4(senstate)
  [limits] -> Actions/3(limits)

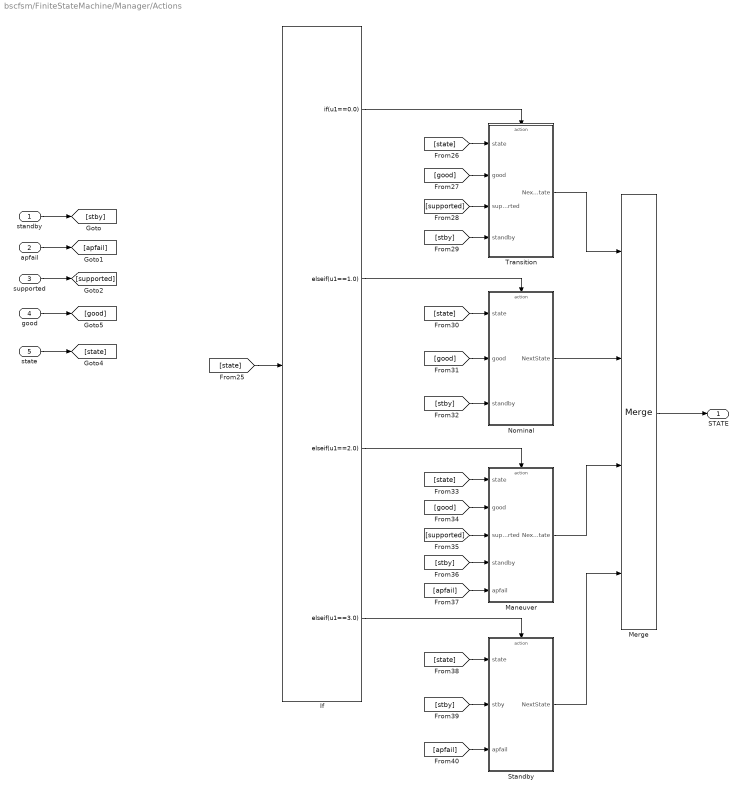
== system bscfsm/FiniteStateMachine/Manager/Actions ==
  standby : Inport
  apfail : Inport  Port=2
  supported : Inport  Port=3
  good : Inport  Port=4
  state : Inport  Port=5
  If : If  IfExpression=u1==0.0  ElseIfExpressions=u1==1.0, u1==2.0, u1==3.0  ShowElse=off
  Maneuver : Subsystem
  Merge : Merge  Inputs=4
  Nominal : Subsystem
  Standby : Subsystem
  Transition : Subsystem
  STATE : Outport
  wires:
  [state] -> If/1
  [state] -> Transition/1(state)
  [apfail] -> Standby/3(apfail)
  [stby] -> Standby/2(stby)
  Standby/1(NextState) -> Merge/4
  [state] -> Standby/1(state)
  Maneuver/1(NextState) -> Merge/3
  Merge/1 -> STATE/1
  Transition/1(NextState) -> Merge/1
  Nominal/1(NextState) -> Merge/2
  If/2 -> Nominal/Action
  [state] -> Nominal/1(state)
  If/3 -> Maneuver/Action
  If/4 -> Standby/Action
  [apfail] -> Maneuver/5(apfail)
  [good] -> Nominal/2(good)
  [stby] -> Nominal/3(standby)
  If/1 -> Transition/Action
  [supported] -> Transition/3(supported)
  [good] -> Transition/2(good)
  [stby] -> Transition/4(standby)
  [state] -> Maneuver/1(state)
  [supported] -> Maneuver/3(supported)
  [good] -> Maneuver/2(good)
  [stby] -> Maneuver/4(standby)
  standby/1 -> [stby]
  supported/1 -> [supported]
  apfail/1 -> [apfail]
  state/1 -> [state]
  good/1 -> [good]

== system bscfsm/FiniteStateMachine/Manager/Output ==
  Newstate : Inport
  Demux : Demux  Outputs=3
  If : If  IfExpression=u1==0.0  ElseIfExpressions=u1==1.0, u1==2.0, u1==3.0  ShowElse=off
  Maneuver : Subsystem
  Merge : Merge  Inputs=4
  Nominal : Subsystem
  Standby : Subsystem
  Transition : Subsystem
  MODE : Outport
  REQUEST : Outport  Port=2
  PULL : Outport  Port=3
  wires:
  Demux/2 -> REQUEST/1  "REQUEST"
  Demux/1 -> MODE/1  "MODE"
  Demux/3 -> PULL/1  "PULL"
  Merge/1 -> Demux/1
  Nominal/1(Output) -> Merge/2
  Maneuver/1(Output) -> Merge/3
  If/2 -> Nominal/Action
  Transition/1(Output) -> Merge/1
  If/3 -> Maneuver/Action
  Standby/1(Output) -> Merge/4
  If/1 -> Transition/Action
  Newstate/1 -> If/1
  If/4 -> Standby/Action

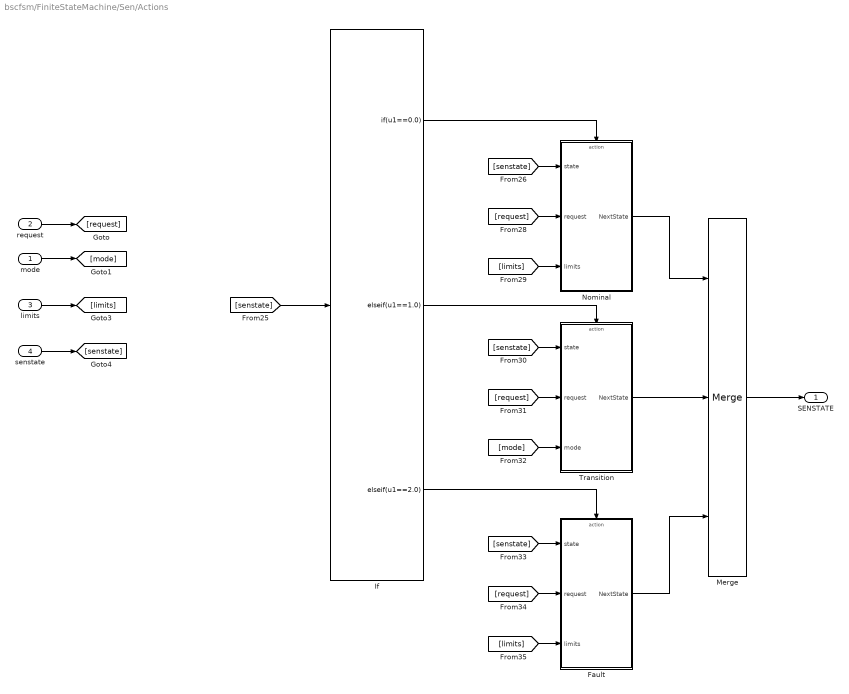
== system bscfsm/FiniteStateMachine/Sen/Actions ==
  mode : Inport
  request : Inport  Port=2
  limits : Inport  Port=3
  senstate : Inport  Port=4
  Fault : Subsystem
  If : If  IfExpression=u1==0.0  ElseIfExpressions=u1==1.0, u1==2.0  ShowElse=off
  Merge : Merge  Inputs=3
  Nominal : Subsystem
  Transition : Subsystem
  SENSTATE : Outport
  wires:
  [senstate] -> If/1
  [senstate] -> Nominal/1(state)
  Fault/1(NextState) -> Merge/3
  Merge/1 -> SENSTATE/1
  Nominal/1(NextState) -> Merge/1
  Transition/1(NextState) -> Merge/2
  If/2 -> Transition/Action
  [senstate] -> Transition/1(state)
  If/3 -> Fault/Action
  [request] -> Transition/2(request)
  [mode] -> Transition/3(mode)
  If/1 -> Nominal/Action
  [request] -> Nominal/2(request)
  [limits] -> Nominal/3(limits)
  [senstate] -> Fault/1(state)
  [limits] -> Fault/3(limits)
  [request] -> Fault/2(request)
  request/1 -> [request]
  mode/1 -> [mode]
  limits/1 -> [limits]
  senstate/1 -> [senstate]

== system bscfsm/FiniteStateMachine/Sen/Output ==
  Newstate : Inport
  Constant12 : Constant  OutDataTypeStr=boolean
  Constant6 : Constant  Value=2
  Constant9 : Constant  Value=0  OutDataTypeStr=boolean
  Relational Operator5 : RelationalOperator  Operator===  OutDataTypeStr=boolean
  Switch2 : Switch  Criteria=u2 ~= 0
  Good : Outport
  wires:
  Constant6/1 -> Relational Operator5/2
  Relational Operator5/1 -> Switch2/2
  Constant9/1 -> Switch2/1
  Constant12/1 -> Switch2/3
  Switch2/1 -> Good/1
  Newstate/1 -> Relational Operator5/1

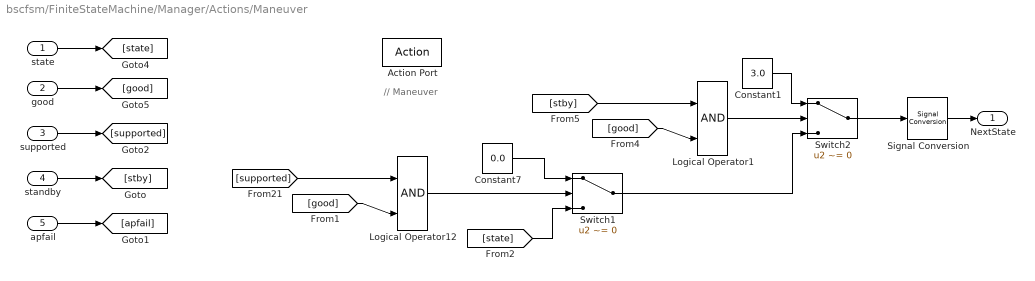
== system bscfsm/FiniteStateMachine/Manager/Actions/Maneuver ==
  note: // Maneuver
  state : Inport
  good : Inport  Port=2
  supported : Inport  Port=3
  standby : Inport  Port=4
  apfail : Inport  Port=5
  Action Port : ActionPort  ActionType=elseif
  Constant1 : Constant  Value=3.0
  Constant7 : Constant  Value=0.0
  Logical Operator1 : Logic  IconShape=distinctive  AllPortsSameDT=off  OutDataTypeStr=boolean
  Logical Operator12 : Logic  IconShape=distinctive  AllPortsSameDT=off  OutDataTypeStr=boolean
  Signal Conversion : SignalConversion  OverrideOpt=off
  Switch1 : Switch  Criteria=u2 ~= 0
  Switch2 : Switch  Criteria=u2 ~= 0
  NextState : Outport
  wires:
  [supported] -> Logical Operator12/1
  Logical Operator12/1 -> Switch1/2
  [state] -> Switch1/3
  Constant7/1 -> Switch1/1
  Logical Operator1/1 -> Switch2/2
  Constant1/1 -> Switch2/1
  Switch2/1 -> Signal Conversion/1
  Signal Conversion/1 -> NextState/1
  standby/1 -> [stby]
  supported/1 -> [supported]
  apfail/1 -> [apfail]
  state/1 -> [state]
  good/1 -> [good]
  [good] -> Logical Operator12/2
  [stby] -> Logical Operator1/1
  [good] -> Logical Operator1/2
  Switch1/1 -> Switch2/3

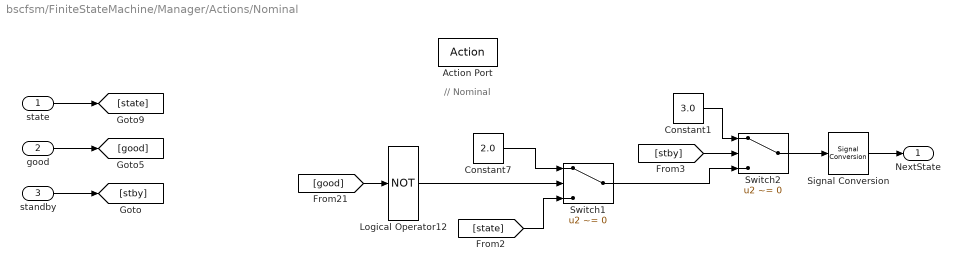
== system bscfsm/FiniteStateMachine/Manager/Actions/Nominal ==
  note: // Nominal
  state : Inport
  good : Inport  Port=2
  standby : Inport  Port=3
  Action Port : ActionPort  ActionType=elseif
  Constant1 : Constant  Value=3.0
  Constant7 : Constant  Value=2.0
  Logical Operator12 : Logic  Operator=NOT  IconShape=distinctive  AllPortsSameDT=off  OutDataTypeStr=boolean
  Signal Conversion : SignalConversion  OverrideOpt=off
  Switch1 : Switch  Criteria=u2 ~= 0
  Switch2 : Switch  Criteria=u2 ~= 0
  NextState : Outport
  wires:
  Signal Conversion/1 -> NextState/1
  Switch2/1 -> Signal Conversion/1
  Switch1/1 -> Switch2/3
  Constant1/1 -> Switch2/1
  [stby] -> Switch2/2
  standby/1 -> [stby]
  Constant7/1 -> Switch1/1
  [state] -> Switch1/3
  Logical Operator12/1 -> Switch1/2
  [good] -> Logical Operator12/1
  good/1 -> [good]
  state/1 -> [state]

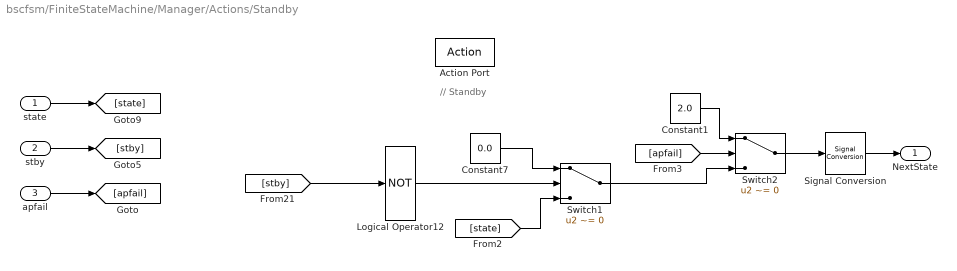
== system bscfsm/FiniteStateMachine/Manager/Actions/Standby ==
  note: // Standby
  state : Inport
  stby : Inport  Port=2
  apfail : Inport  Port=3
  Action Port : ActionPort  ActionType=elseif
  Constant1 : Constant  Value=2.0
  Constant7 : Constant  Value=0.0
  Logical Operator12 : Logic  Operator=NOT  IconShape=distinctive  AllPortsSameDT=off  OutDataTypeStr=boolean
  Signal Conversion : SignalConversion  OverrideOpt=off
  Switch1 : Switch  Criteria=u2 ~= 0
  Switch2 : Switch  Criteria=u2 ~= 0
  NextState : Outport
  wires:
  Signal Conversion/1 -> NextState/1
  Switch2/1 -> Signal Conversion/1
  Switch1/1 -> Switch2/3
  Constant1/1 -> Switch2/1
  [apfail] -> Switch2/2
  apfail/1 -> [apfail]
  Constant7/1 -> Switch1/1
  [state] -> Switch1/3
  Logical Operator12/1 -> Switch1/2
  [stby] -> Logical Operator12/1
  stby/1 -> [stby]
  state/1 -> [state]

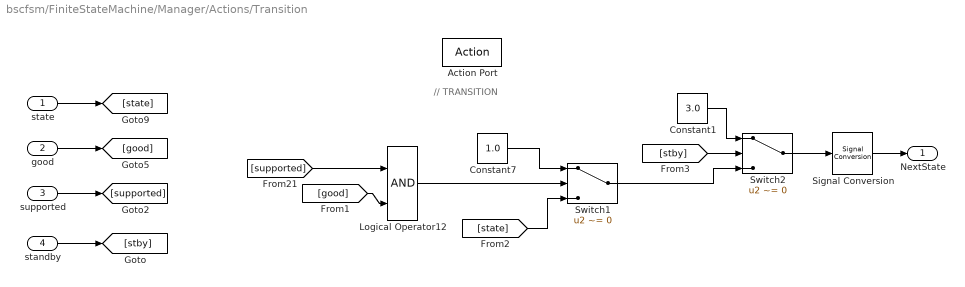
== system bscfsm/FiniteStateMachine/Manager/Actions/Transition ==
  note: // TRANSITION
  state : Inport
  good : Inport  Port=2
  supported : Inport  Port=3
  standby : Inport  Port=4
  Action Port : ActionPort  ActionType=then
  Constant1 : Constant  Value=3.0
  Constant7 : Constant  Value=1.0
  Logical Operator12 : Logic  IconShape=distinctive  AllPortsSameDT=off  OutDataTypeStr=boolean
  Signal Conversion : SignalConversion  OverrideOpt=off
  Switch1 : Switch  Criteria=u2 ~= 0
  Switch2 : Switch  Criteria=u2 ~= 0
  NextState : Outport
  wires:
  state/1 -> [state]
  good/1 -> [good]
  supported/1 -> [supported]
  [supported] -> Logical Operator12/1
  [good] -> Logical Operator12/2
  Logical Operator12/1 -> Switch1/2
  [state] -> Switch1/3
  Constant7/1 -> Switch1/1
  standby/1 -> [stby]
  [stby] -> Switch2/2
  Constant1/1 -> Switch2/1
  Switch1/1 -> Switch2/3
  Switch2/1 -> Signal Conversion/1
  Signal Conversion/1 -> NextState/1

== system bscfsm/FiniteStateMachine/Manager/Output/Maneuver ==
  note: // Maneuver
  note: PULL
  Action Port : ActionPort  ActionType=elseif
  Constant10 : Constant  Value=0  OutDataTypeStr=boolean
  Constant11 : Constant  OutDataTypeStr=boolean
  Constant9 : Constant  OutDataTypeStr=boolean
  Mux2 : Mux  Inputs=3
  Output : Outport
  wires:
  Mux2/1 -> Output/1
  Constant10/1 -> Mux2/2
  Constant11/1 -> Mux2/3
  Constant9/1 -> Mux2/1

== system bscfsm/FiniteStateMachine/Manager/Output/Nominal ==
  note: // Nominal
  note: OPS
  Action Port : ActionPort  ActionType=elseif
  Constant3 : Constant  OutDataTypeStr=boolean
  Constant4 : Constant  OutDataTypeStr=boolean
  Constant5 : Constant  Value=0  OutDataTypeStr=boolean
  Mux1 : Mux  Inputs=3
  Output : Outport
  wires:
  Constant5/1 -> Mux1/3
  Constant4/1 -> Mux1/2
  Constant3/1 -> Mux1/1
  Mux1/1 -> Output/1

== system bscfsm/FiniteStateMachine/Manager/Output/Standby ==
  note: PULL
  note: // Standby
  Action Port : ActionPort  ActionType=elseif
  Constant1 : Constant  Value=0  OutDataTypeStr=boolean
  Constant11 : Constant  Value=0  OutDataTypeStr=boolean
  Constant9 : Constant  OutDataTypeStr=boolean
  Mux2 : Mux  Inputs=3
  Output : Outport
  wires:
  Constant9/1 -> Mux2/1
  Constant11/1 -> Mux2/3
  Constant1/1 -> Mux2/2
  Mux2/1 -> Output/1

== system bscfsm/FiniteStateMachine/Manager/Output/Transition ==
  note: // TRANSITION
  note: TRANSITION
  Action Port : ActionPort  ActionType=then
  Constant16 : Constant  Value=0  OutDataTypeStr=boolean
  Constant17 : Constant  OutDataTypeStr=boolean
  Constant18 : Constant  Value=0  OutDataTypeStr=boolean
  Mux4 : Mux  Inputs=3
  Output : Outport
  wires:
  Mux4/1 -> Output/1
  Constant17/1 -> Mux4/2
  Constant16/1 -> Mux4/1
  Constant18/1 -> Mux4/3

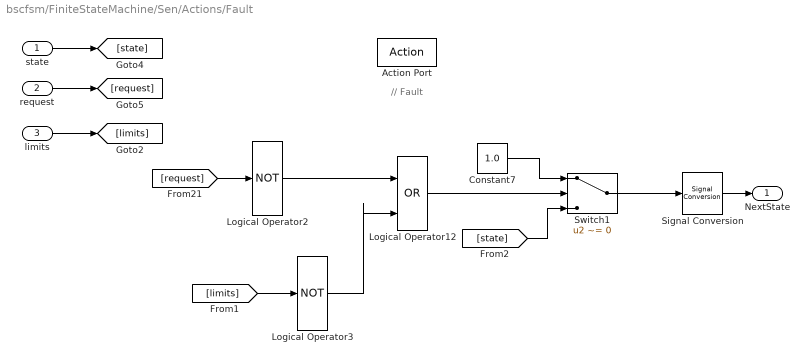
== system bscfsm/FiniteStateMachine/Sen/Actions/Fault ==
  note: // Fault
  state : Inport
  request : Inport  Port=2
  limits : Inport  Port=3
  Action Port : ActionPort  ActionType=elseif
  Constant7 : Constant  Value=1.0
  Logical Operator12 : Logic  Operator=OR  IconShape=distinctive  AllPortsSameDT=off  OutDataTypeStr=boolean
  Logical Operator2 : Logic  Operator=NOT  IconShape=distinctive  AllPortsSameDT=off  OutDataTypeStr=boolean
  Logical Operator3 : Logic  Operator=NOT  IconShape=distinctive  AllPortsSameDT=off  OutDataTypeStr=boolean
  Signal Conversion : SignalConversion  OverrideOpt=off
  Switch1 : Switch  Criteria=u2 ~= 0
  NextState : Outport
  wires:
  [request] -> Logical Operator2/1
  Logical Operator12/1 -> Switch1/2
  [state] -> Switch1/3
  Constant7/1 -> Switch1/1
  Switch1/1 -> Signal Conversion/1
  Signal Conversion/1 -> NextState/1
  limits/1 -> [limits]
  state/1 -> [state]
  request/1 -> [request]
  Logical Operator2/1 -> Logical Operator12/1
  [limits] -> Logical Operator3/1
  Logical Operator3/1 -> Logical Operator12/2

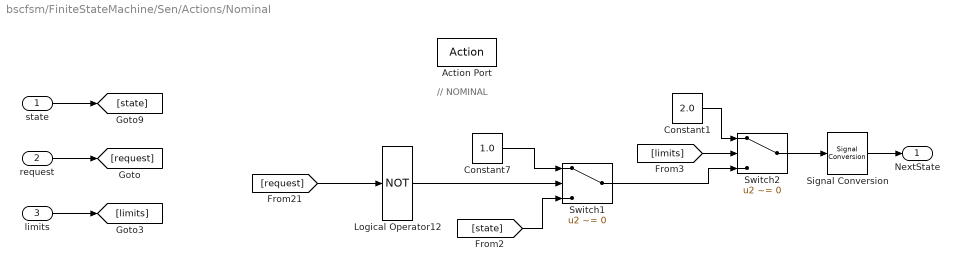
== system bscfsm/FiniteStateMachine/Sen/Actions/Nominal ==
  note: // NOMINAL
  state : Inport
  request : Inport  Port=2
  limits : Inport  Port=3
  Action Port : ActionPort  ActionType=then
  Constant1 : Constant  Value=2.0
  Constant7 : Constant  Value=1.0
  Logical Operator12 : Logic  Operator=NOT  IconShape=distinctive  AllPortsSameDT=off  OutDataTypeStr=boolean
  Signal Conversion : SignalConversion  OverrideOpt=off
  Switch1 : Switch  Criteria=u2 ~= 0
  Switch2 : Switch  Criteria=u2 ~= 0
  NextState : Outport
  wires:
  state/1 -> [state]
  [request] -> Logical Operator12/1
  Logical Operator12/1 -> Switch1/2
  [state] -> Switch1/3
  Constant7/1 -> Switch1/1
  [limits] -> Switch2/2
  Constant1/1 -> Switch2/1
  Switch1/1 -> Switch2/3
  Switch2/1 -> Signal Conversion/1
  Signal Conversion/1 -> NextState/1
  request/1 -> [request]
  limits/1 -> [limits]

== system bscfsm/FiniteStateMachine/Sen/Actions/Transition ==
  note: // Transition
  state : Inport
  request : Inport  Port=2
  mode : Inport  Port=3
  Action Port : ActionPort  ActionType=elseif
  Constant7 : Constant  Value=0.0
  Logical Operator12 : Logic  IconShape=distinctive  AllPortsSameDT=off  OutDataTypeStr=boolean
  Signal Conversion : SignalConversion  OverrideOpt=off
  Switch1 : Switch  Criteria=u2 ~= 0
  NextState : Outport
  wires:
  Signal Conversion/1 -> NextState/1
  Switch1/1 -> Signal Conversion/1
  mode/1 -> [mode]
  Constant7/1 -> Switch1/1
  [state] -> Switch1/3
  Logical Operator12/1 -> Switch1/2
  [request] -> Logical Operator12/1
  request/1 -> [request]
  state/1 -> [state]
  [mode] -> Logical Operator12/2
